simulink model "tx"  (R2019a)
settings: Solver=VariableStepAuto  StartTime=0.0  StopTime=10  RelTol=1e-3
undefined symbols (not defined in the file): fdesignblkfcn, gcbh
libraries: commnoisgen2 x1, dspobslib x1
(part 1 of 2)
settings Model: Creator=vicda  LastModifiedBy=vicda

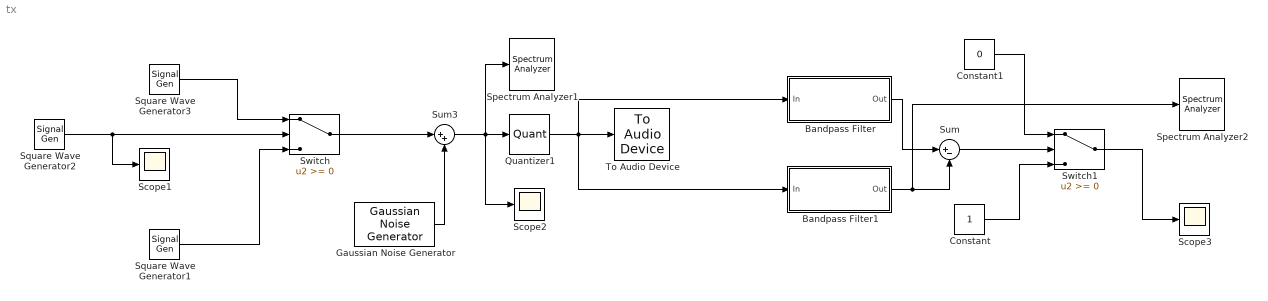
== system tx ==
  Bandpass Filter : Subsystem  DialogController=fdesignblkfcn  InitFcn=fdesignblkfcn(gcbh, {'InitFcn'});  mask(Bandpass Filter){}
      mask help: Design a bandpass filter
      settings: CopyFcn=fdesignblkfcn(gcbh, {'CopyFcn'});
      mask Help: helpview(mapfilelocation('dsp'), 'dspbandpassfilter');
      mask Display: disp('Bandpass');
  Bandpass Filter1 : Subsystem  DialogController=fdesignblkfcn  InitFcn=fdesignblkfcn(gcbh, {'InitFcn'});  mask(Bandpass Filter){}
      mask help: Design a bandpass filter
      settings: CopyFcn=fdesignblkfcn(gcbh, {'CopyFcn'});
      mask Help: helpview(mapfilelocation('dsp'), 'dspbandpassfilter');
      mask Display: disp('Bandpass');
  Constant : Constant
  Constant1 : Constant  Value=0
  Gaussian Noise Generator : commnoisgen2/Gaussian Noise Generator  m=0  d=0  s=200  Ts=1e-4  frameBased=off  sampPerFrame=1  orient=off  outDataType=double
      settings: SourceProductName=Communications Toolbox  SourceProductBaseCode=CM
  Quantizer1 : Quantizer  QuantizationInterval=0.01  LinearizeAsGain=off  SampleTime=1/44100
  Scope1 : Scope
  Scope2 : Scope
  Scope3 : Scope
  Spectrum Analyzer1 : SpectrumAnalyzer
  Spectrum Analyzer2 : SpectrumAnalyzer
  Square Wave Generator1 : SignalGenerator  Amplitude=0.5  Frequency=200
  Square Wave Generator2 : SignalGenerator  WaveForm=square  Amplitude=0.5  Frequency=3
  Square Wave Generator3 : SignalGenerator  Amplitude=0.5  Frequency=400
  Sum : Sum  Inputs=|+-
  Sum3 : Sum  Inputs=|++  SampleTime=1e-4
  Switch : Switch
  Switch1 : Switch
  To Audio Device : dspobslib/To Audio Device  deviceName=Default  inheritSampleRate=off  sampleRate=44100  deviceDatatype=Determine from input data type  autoBufferSize=on  bufferSize=4096  queueDuration=1.0  defaultOutputChannelMapping=on  outputChannelMapping=1:2  outputNumUnderrunSamples=off
      settings: SourceProductName=DSP System Toolbox  SourceProductBaseCode=DS
  wires:
  Square Wave Generator3/1 -> Switch/1
  Square Wave Generator1/1 -> Switch/3
  Square Wave Generator2/1 -> Scope1/1, Switch/2
  Gaussian Noise Generator/1 -> Sum3/2
  Switch/1 -> Sum3/1
  Sum3/1 -> Scope2/1, Spectrum Analyzer1/1, Quantizer1/1
  Bandpass Filter/1(Out) -> Sum/1
  Bandpass Filter1/1(Out) -> Spectrum Analyzer2/1, Sum/2
  Switch1/1 -> Scope3/1
  Quantizer1/1 -> Bandpass Filter1/1(In), Bandpass Filter/1(In), To Audio Device/1
  Constant/1 -> Switch1/3
  Sum/1 -> Switch1/2
  Constant1/1 -> Switch1/1

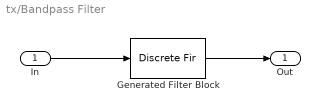
== system tx/Bandpass Filter ==
  In : Inport
  Generated Filter Block : DiscreteFir  Tag=BlockMethodSubSystem  Coefficients=[0.000900824085080897344 1.70374766476774023e-05 1.67118107804677032e-05 1.7208674576677397e-05 1.68061361482797853e-05 1.72335492297530021e-05 1.67472279588890775e-05 1.7106611413632419e-05 1.65281181264917984e-05 1.68253657554211103e-05 1.6144671941647668e-05 1.63986051431437531e-05 1.56020849602289333e-05 1.58815661131654932e-05 1.49429886802225371e-05 1.57422490407198084e-05 1.63082228054177046e-05 1.46451548477439814e-05 1.44777921974255418e-05 1.42621803858281482e-05 1.37038102221476209e-05 1.35412393777197384e-05 1.28558168138453869e-05 1.26854308383028778e-05 1.19048288668445988e-05 1.17044706158500773e-05 1.08317826751418112e-05 1.05952575656065003e-05 9.62766702701219144e-06 9.38627399215286734e-06 8.33535093183962548e-06 8.39457007291986076e-06 7.57738685762377427e-06 6.88111520118553626e-06 6.13348165500967636e-06 5.70729568384804355e-06 4.82521695077382882e-06 4.43686085584669987e-06 3.51564911640607578e-06 3.14202168090981209e-06 2.19448454716981642e-06 1.82439132594819624e-06 8.47772812189459893e-07 4.73414621392199107e-07 -5.36868816449864554e-07 -8.97145978939035103e-07 -1.91410355055733877e-06 -2.03977029069430608e-06 -3.02882678418492368e-06 -3.4467320169163148e-06 -4.26740955954108513e-06 -4.59190152297516557e-06 -5.41773134395693093e-06 -5.67686805051312044e-06 -6.46598974101135655e-06 -6.66383300262452048e-06 -7.40742249081324106e-06 -7.54829667115011933e-06 -8.25040244441580233e-06 -8.3437241521510698e-06 -9.01081571075366006e-06 -9.04773678298681754e-06 -9.64379987782851191e-06 -9.46803953097799002e-06 -1.00631542920967196e-05 -9.95486230554809906e-06 -1.03661602823501521e-05 -1.01870985269719976e-05 -1.05286548363980968e-05 -1.0258859946671783e-05 -1.05149647763509192e-05 -1.01522233976576119e-05 -1.03188228588191062e-05 -9.86662439063389941e-06 -9.95088104544005272e-06 -9.4221442338361704e-06 -9.43401385041918884e-06 -8.82785524957286488e-06 -8.7276370367814389e-06 -7.94396202684864716e-06 -7.84442834166879013e-06 -7.0251881113882501e-06 -6.77280600066881757e-06 -5.89575901882328102e-06 -5.55993047857041966e-06 -4.60364499401798993e-06 -4.18530856605506003e-06 -3.15002571273331582e-06 -2.65188012228451293e-06 -1.54516474230360652e-06 -9.80066849955401991e-07 1.7967649056918264e-07 7.96971514754451354e-07 2.00506574197666012e-06 2.71412913141716276e-06 4.02136681356421791e-06 4.69881945362445128e-06 6.04613397481995607e-06 6.79739807091543288e-06 8.15258976134272065e-06 8.93672124865517101e-06 1.03087072545784671e-05 1.1113904856707886e-05 1.24962430036119941e-05 1.33123961063842623e-05 1.46916698223896643e-05 1.54994177995888523e-05 1.68514808715532075e-05 1.76308026841396747e-05 1.89477269143586285e-05 1.97344588308815847e-05 2.10263136125181686e-05 2.17057191245127691e-05 2.29619714200782199e-05 2.35920361997711677e-05 2.47610910756091741e-05 2.53185029483718373e-05 2.63967211303208589e-05 2.6864970397596946e-05 2.78414940715384761e-05 2.8206345925894721e-05 2.9063866697487937e-05 2.93022725453909172e-05 3.00140198091592781e-05 3.01042420461427674e-05 3.06639835642384109e-05 3.06370766557709489e-05 3.10258393292920038e-05 3.07898697527199654e-05 3.10251153906766775e-05 3.06019622326543419e-05 3.06340977504268716e-05 3.00132860841951371e-05 2.9833279449923214e-05 2.90013410428752172e-05 2.85999623718744943e-05 2.75457360204659505e-05 2.69085736973092432e-05 2.56121751307388477e-05 2.47167087797619178e-05 2.31616249796706133e-05 2.20108520478125552e-05 2.02263610255904239e-05 1.87876877542377104e-05 1.67145599137672905e-05 1.50224034239191144e-05 1.2663376817654442e-05 1.06854031174606059e-05 8.04273704362533891e-06 5.77468858841453502e-06 2.84587344431125322e-06 2.88280445415243884e-07 -2.92709246703089319e-06 -5.77773617204085758e-06 -9.28817701458645693e-06 -1.24417437396681305e-05 -1.62500945037143043e-05 -1.96871786435146977e-05 -2.37618173798084418e-05 -2.75125040327304192e-05 -3.18740145369175547e-05 -3.58925891991898052e-05 -4.05416073076347947e-05 -4.48354743750740666e-05 ...(+38029 chars)]  InputProcessing=Columns as channels (frame based)
  Out : Outport
  wires:
  In/1 -> Generated Filter Block/1
  Generated Filter Block/1 -> Out/1
